simulink model "TableDeMiaxage"  (R2019a)
settings: Solver=VariableStepAuto  StartTime=0.0  StopTime=180  RelTol=1e-3
undefined symbols (not defined in the file): fdesignblkfcn, gcbh
libraries: dspvision x3, dspobslib x2, dspsrcs4 x1
settings Model: Creator=Ahmed  LastModifiedBy=shse

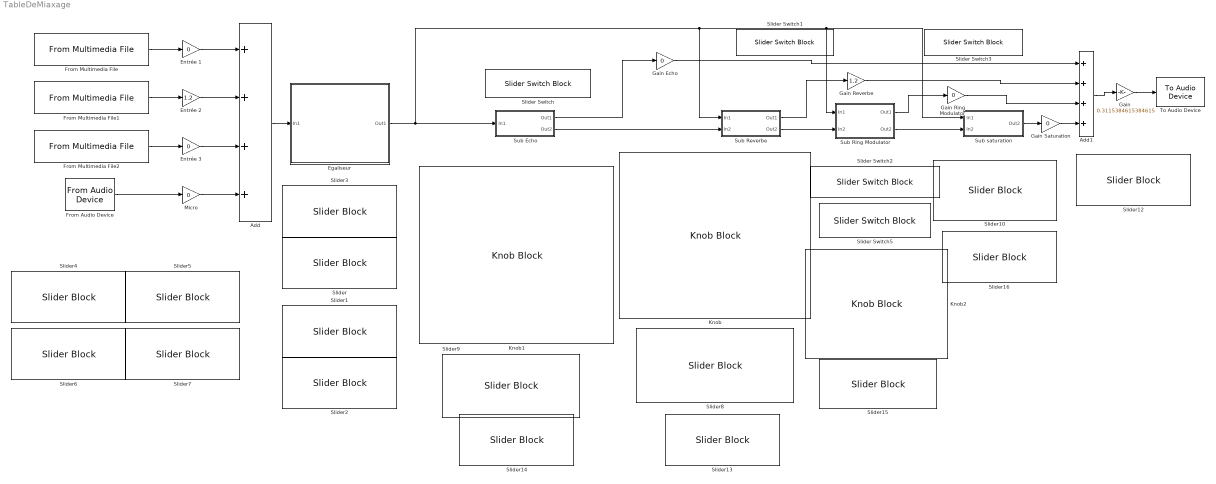
== system TableDeMiaxage ==
  Add : Sum  Inputs=++++
  Add1 : Sum  Inputs=++++
  Egaliseur : Subsystem
  Entrée 1 : Gain  Gain=0
  Entrée 2 : Gain  Gain=1.2
  Entrée 3 : Gain  Gain=0
  From Audio Device : dspobslib/From Audio Device  deviceName="Microphone (AT2020 USB               )"  numChannels=2  sampleRate=48000  deviceDatatype=Determine from output data type  autoBufferSize=on  bufferSize=4096  queueDuration=1.0  frameSize=1024  outputDatatype=double  defaultInputChannelMapping=on  inputChannelMapping=1:2  outputNumOverrunSamples=off  OutputFrames=on
      settings: SourceProductName=DSP System Toolbox  SourceProductBaseCode=DS
  From Multimedia File : dspvision/From Multimedia File  inputFilename=C:\Users\Ahmed\Nextcloud\L3\LU3EE105\Audio\Documents de TP et projet-20191118\Projet\because.wav  readRange=[1 Inf]  loop=on  numPlays=inf  outputStreams=Audio only  videoDataType=single  audioDataType=double  inheritSampleTime=on  userDefinedSampleTime=1/30  noAudioOutput=off  isIntensityVideo=off  fourcc=RGB  colorVideoFormat=Separate color signals  outputEOF=off  dataOrg=Column-major  audioFrameSize=1024  computeAudioFrameSize=off  outSamplingMode=Sample based
      settings: SourceProductName=DSP System Toolbox  SourceProductBaseCode=DS
  From Multimedia File1 : dspvision/From Multimedia File  inputFilename=C:\Users\Ahmed\Nextcloud\L3\LU3EE105\Audio\Documents de TP et projet-20191118\Projet\superstition.wav  readRange=[1 Inf]  loop=on  numPlays=inf  outputStreams=Audio only  videoDataType=single  audioDataType=double  inheritSampleTime=on  userDefinedSampleTime=1/30  noAudioOutput=off  isIntensityVideo=off  fourcc=RGB  colorVideoFormat=Separate color signals  outputEOF=off  dataOrg=Column-major  audioFrameSize=1024  computeAudioFrameSize=off  outSamplingMode=Sample based
      settings: SourceProductName=DSP System Toolbox  SourceProductBaseCode=DS
  From Multimedia File2 : dspvision/From Multimedia File  inputFilename=C:\Users\Ahmed\Nextcloud\L3\LU3EE105\Audio\Documents de TP et projet-20191118\Projet\tchai.wav  readRange=[1 Inf]  loop=on  numPlays=inf  outputStreams=Audio only  videoDataType=single  audioDataType=double  inheritSampleTime=on  userDefinedSampleTime=1/30  noAudioOutput=off  isIntensityVideo=off  fourcc=RGB  colorVideoFormat=Separate color signals  outputEOF=off  dataOrg=Column-major  audioFrameSize=1024  computeAudioFrameSize=off  outSamplingMode=Sample based
      settings: SourceProductName=DSP System Toolbox  SourceProductBaseCode=DS
  Gain : Gain  Gain=0.3115384615384615
  Gain Echo : Gain  Gain=0
  Gain Reverbe : Gain  Gain=1.2
  Gain Ring Modulator : Gain  Gain=0
  Gain Saturation : Gain  Gain=0
  Knob : KnobBlock  ScaleMax=48000
  Knob1 : KnobBlock  ScaleMax=48000
  Knob2 : KnobBlock  ScaleMin=100  ScaleMax=2000
  Micro : Gain  Gain=0
  Slider{,1..7} (8 alike) : SliderBlock  ScaleMax=1.2
  Slider Switch{,1..3,5} (5 alike) : SliderSwitchBlock
  Slider10 : SliderBlock  ScaleMax=1.5
  Slider12 : SliderBlock  ScaleMax=1.5
  Slider{13..16} (4 alike) : SliderBlock  ScaleMax=2
  Slider8 : SliderBlock  ScaleMax=1
  Slider9 : SliderBlock  ScaleMax=1
  Sub Echo : Subsystem
  Sub Reverbe : Subsystem
  Sub Ring Modulator : Subsystem
  Sub saturation : Subsystem
  To Audio Device : dspobslib/To Audio Device  deviceName=Default  inheritSampleRate=on  sampleRate=44100  deviceDatatype=Determine from input data type  autoBufferSize=on  bufferSize=4096  queueDuration=1.0  defaultOutputChannelMapping=on  outputChannelMapping=1:2  outputNumUnderrunSamples=off
      settings: SourceProductName=DSP System Toolbox  SourceProductBaseCode=DS
  wires:
  From Multimedia File/1 -> Entrée 1/1
  From Multimedia File1/1 -> Entrée 2/1
  From Multimedia File2/1 -> Entrée 3/1
  From Audio Device/1 -> Micro/1
  Micro/1 -> Add/4
  Entrée 3/1 -> Add/3
  Entrée 2/1 -> Add/2
  Entrée 1/1 -> Add/1
  Add/1 -> Egaliseur/1(In1)
  Add1/1 -> Gain/1
  Sub Reverbe/2(Out2) -> Sub Ring Modulator/2(In2)
  Sub Reverbe/1(Out1) -> Gain Reverbe/1
  Sub Echo/2(Out2) -> Sub Reverbe/2(In2)
  Egaliseur/1(Out1) -> Sub Reverbe/1(In1), Sub Ring Modulator/1(In1), Sub saturation/1(In1), Sub Echo/1(In1)
  Sub Echo/1(Out1) -> Gain Echo/1
  Gain/1 -> To Audio Device/1
  Sub saturation/1(Out2) -> Gain Saturation/1
  Sub Ring Modulator/2(Out2) -> Sub saturation/2(In2)
  Sub Ring Modulator/1(Out1) -> Gain Ring Modulator/1
  Gain Echo/1 -> Add1/1
  Gain Reverbe/1 -> Add1/2
  Gain Ring Modulator/1 -> Add1/3
  Gain Saturation/1 -> Add1/4

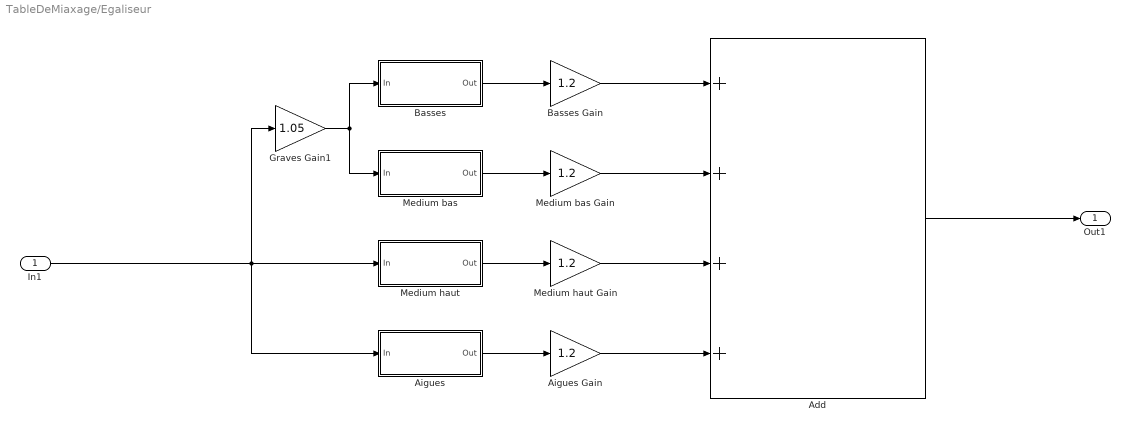
== system TableDeMiaxage/Egaliseur ==
  In1 : Inport
  Add : Sum  Inputs=++++
  Aigues : Subsystem  DialogController=fdesignblkfcn  InitFcn=fdesignblkfcn(gcbh, {'InitFcn'});  mask(Highpass Filter){}
      mask help: Design a highpass filter
      settings: CopyFcn=fdesignblkfcn(gcbh, {'CopyFcn'});
      mask Help: helpview(mapfilelocation('dsp'), 'dsphighpassfilter');
      mask Display: disp('Highpass')
  Aigues Gain : Gain  Gain=1.2
  Basses : Subsystem  DialogController=fdesignblkfcn  InitFcn=fdesignblkfcn(gcbh, {'InitFcn'});  mask(Lowpass Filter){}
      mask help: Design a lowpass filter
      settings: CopyFcn=fdesignblkfcn(gcbh, {'CopyFcn'});
      mask Help: helpview(mapfilelocation('dsp'), 'dsplowpassfilter');
      mask Display: disp('Lowpass')
  Basses Gain : Gain  Gain=1.2
  Graves Gain1 : Gain  Gain=1.05
  Medium bas : Subsystem  DialogController=fdesignblkfcn  InitFcn=fdesignblkfcn(gcbh, {'InitFcn'});  mask(Bandpass Filter){}
      mask help: Design a bandpass filter
      settings: CopyFcn=fdesignblkfcn(gcbh, {'CopyFcn'});
      mask Help: helpview(mapfilelocation('dsp'), 'dspbandpassfilter');
      mask Display: disp('Bandpass');
  Medium bas Gain : Gain  Gain=1.2
  Medium haut : Subsystem  DialogController=fdesignblkfcn  InitFcn=fdesignblkfcn(gcbh, {'InitFcn'});  mask(Bandpass Filter){}
      mask help: Design a bandpass filter
      settings: CopyFcn=fdesignblkfcn(gcbh, {'CopyFcn'});
      mask Help: helpview(mapfilelocation('dsp'), 'dspbandpassfilter');
      mask Display: disp('Bandpass');
  Medium haut Gain : Gain  Gain=1.2
  Out1 : Outport
  wires:
  Graves Gain1/1 -> Basses/1(In), Medium bas/1(In)
  Add/1 -> Out1/1
  Aigues Gain/1 -> Add/4
  Medium haut Gain/1 -> Add/3
  Medium bas/1(Out) -> Medium bas Gain/1
  Medium bas Gain/1 -> Add/2
  Basses Gain/1 -> Add/1
  Basses/1(Out) -> Basses Gain/1
  In1/1 -> Aigues/1(In), Medium haut/1(In), Graves Gain1/1
  Medium haut/1(Out) -> Medium haut Gain/1
  Aigues/1(Out) -> Aigues Gain/1

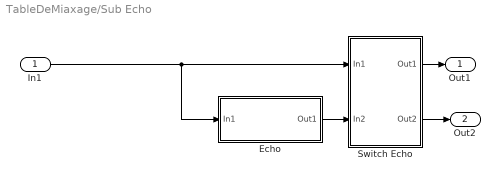
== system TableDeMiaxage/Sub Echo ==
  In1 : Inport
  Echo : Subsystem
  Switch Echo : Subsystem
  Out1 : Outport
  Out2 : Outport  Port=2
  wires:
  Echo/1(Out1) -> Switch Echo/2(In2)
  Switch Echo/1(Out1) -> Out1/1
  In1/1 -> Echo/1(In1), Switch Echo/1(In1)
  Switch Echo/2(Out2) -> Out2/1

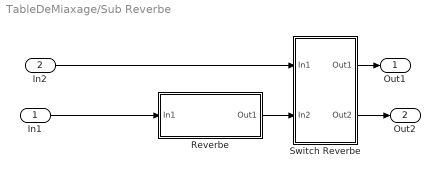
== system TableDeMiaxage/Sub Reverbe ==
  In1 : Inport
  In2 : Inport  Port=2
  Reverbe : Subsystem
  Switch Reverbe : Subsystem
  Out1 : Outport
  Out2 : Outport  Port=2
  wires:
  In1/1 -> Reverbe/1(In1)
  Reverbe/1(Out1) -> Switch Reverbe/2(In2)
  In2/1 -> Switch Reverbe/1(In1)
  Switch Reverbe/2(Out2) -> Out2/1
  Switch Reverbe/1(Out1) -> Out1/1

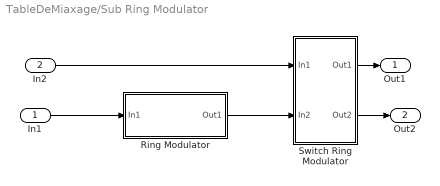
== system TableDeMiaxage/Sub Ring Modulator ==
  In1 : Inport
  In2 : Inport  Port=2
  Ring Modulator : Subsystem
  Switch Ring Modulator : Subsystem
  Out1 : Outport
  Out2 : Outport  Port=2
  wires:
  In1/1 -> Ring Modulator/1(In1)
  Ring Modulator/1(Out1) -> Switch Ring Modulator/2(In2)
  In2/1 -> Switch Ring Modulator/1(In1)
  Switch Ring Modulator/2(Out2) -> Out2/1
  Switch Ring Modulator/1(Out1) -> Out1/1

== system TableDeMiaxage/Sub saturation ==
  In1 : Inport
  In2 : Inport  Port=2
  Switch saturation : Subsystem
  saturation : Subsystem
  Out2 : Outport
  wires:
  In1/1 -> saturation/1(In1)
  saturation/1(Out1) -> Switch saturation/2(In2)
  In2/1 -> Switch saturation/1(In1)
  Switch saturation/1(Out2) -> Out2/1

== system TableDeMiaxage/Egaliseur/Aigues ==
  In : Inport
  Generated Filter Block : DiscreteFir  Tag=BlockMethodSubSystem  Coefficients=[0.0167926706972023297 -0.00307522082859672382 -0.00155836801096264905 0.00678688212494691322 -0.00921947504734154516 0.00716180335937461818 -0.00202417819565003281 -0.00247958884121546579 0.00297471068413305249 0.000980534073277820146 -0.00634024282569068624 0.00870304843048571274 -0.00569033146091242701 -0.000974243416099627264 0.00644942423308224929 -0.00633706852781140001 0.000239642776776960632 0.00749483357856131193 -0.0107451066385319625 0.00631082658742477751 0.00317079948780857714 -0.0107615026768319855 0.0101264166919688165 -0.000871435749622451617 -0.0105995290115455873 0.0152814722852097698 -0.00843240688530845495 -0.00602945332444454647 0.0174768179112361685 -0.016173414015238835 0.00118274129148582654 0.0175174930605758797 -0.0252362821856293232 0.0134963666514811807 0.0120367581497580443 -0.0332563662689180084 0.0313194480469127026 -0.00133439181794675599 -0.0402321887557888502 0.0620015888628606057 -0.0357204359625284198 -0.044553870224684676 0.154599277267642304 -0.249627721101705446 0.287093803988040797 -0.249627721101705446 0.154599277267642304 -0.044553870224684676 -0.0357204359625284198 0.0620015888628606057 -0.0402321887557888502 -0.00133439181794675599 0.0313194480469127026 -0.0332563662689180084 0.0120367581497580443 0.0134963666514811807 -0.0252362821856293232 0.0175174930605758797 0.00118274129148582654 -0.016173414015238835 0.0174768179112361685 -0.00602945332444454647 -0.00843240688530845495 0.0152814722852097698 -0.0105995290115455873 -0.000871435749622451617 0.0101264166919688165 -0.0107615026768319855 0.00317079948780857714 0.00631082658742477751 -0.0107451066385319625 0.00749483357856131193 0.000239642776776960632 -0.00633706852781140001 0.00644942423308224929 -0.000974243416099627264 -0.00569033146091242701 0.00870304843048571274 -0.00634024282569068624 0.000980534073277820146 0.00297471068413305249 -0.00247958884121546579 -0.00202417819565003281 0.00716180335937461818 -0.00921947504734154516 0.00678688212494691322 -0.00155836801096264905 -0.00307522082859672382 0.0167926706972023297]  InputProcessing=Columns as channels (frame based)
  Out : Outport
  wires:
  In/1 -> Generated Filter Block/1
  Generated Filter Block/1 -> Out/1

== system TableDeMiaxage/Egaliseur/Basses ==
  In : Inport
  Generated Filter Block : DiscreteFir  Tag=BlockMethodSubSystem  Coefficients=[-0.0153884254991570896 0.000266804767962262673 0.000327964912984287542 0.000425773956292074178 0.000562470431597255683 0.000729675436245145743 0.000928098732682747078 0.00114757496934848988 0.0013874893535819144 0.00163674485373585228 0.00189397943095723415 0.00214911176559310756 0.00239127376957799917 0.00261871580170263676 0.00282463549794394458 0.00299796194879956577 0.00313700441606081177 0.00323118901775356227 0.00328059593937512052 0.0032762274085140616 0.00321999924325729308 0.00310514488595467486 0.00293597620135533548 0.00271021313991444326 0.00243244432834343769 0.00210285539361005757 0.00173075814627612814 0.00131794874767348713 0.000876458309185095593 0.000409765769008486587 -6.78152181175429349e-05 -0.00055107827022111359 -0.00102452357018295213 -0.00148228311788735465 -0.00190917788438955548 -0.00229835807769330699 -0.00263554870259227183 -0.00291558267477844222 -0.00312595002418917817 -0.00326368850063736733 -0.0033181487660765268 -0.00329019210437426091 -0.00317265655073278429 -0.00297008708884775961 -0.00267912961982578503 -0.00230819118685900767 -0.00185871380492080222 -0.00134285673590555732 -0.000766282213175846516 -0.000143639886938228738 0.000515387431471188277 0.00119186250405529915 0.00187540925341580437 0.00254498623467350367 0.00318890021840806609 0.00378542058067834163 0.00432300298736445088 0.00478127017511513746 0.00515003046032541049 0.00541280250324055381 0.00555799365296140262 0.00557670671392240021 0.00546500919878054655 0.00521345698067954538 0.0048255975064855107 0.00429822188412450328 0.00364138491650149547 0.00285830087950445259 0.00196522256851390346 0.000971608832914958248 -0.000117014335600230956 -0.00121216225006984778 -0.00238215104275762242 -0.00356276040555317426 -0.00472456049283136344 -0.0058457030770970005 -0.00689286435319730502 -0.00784296295490719345 -0.00866238471873602076 -0.00932881033341804826 -0.00981062820326479915 -0.0100871412549760533 -0.0101477740694355528 -0.00995366092214836767 -0.00949962887211590855 -0.00877727431061372382 -0.00777478005111272019 -0.00649472069378163788 -0.0049340887119306712 -0.0031050204118294694 -0.0010140823683356785 0.0013172912006325472 0.00387347512217753364 0.00662624416734313923 0.00954783933336443569 0.0126033841210471554 0.015761493515271157 0.0189793379213840825 0.022221591185954695 0.025441734970274868 0.0286029070172382494 0.0316580472453209458 0.0345709721826798211 0.0372966552097049875 0.039801977564689818 0.0420483051028727392 0.0440079277575662273 0.0456487202321445365 0.0469517485160680023 0.0478939985283200892 0.0484669205309821716 0.0486571254135078901 0.0484669205309821716 0.0478939985283200892 0.0469517485160680023 0.0456487202321445365 0.0440079277575662273 0.0420483051028727392 0.039801977564689818 0.0372966552097049875 0.0345709721826798211 0.0316580472453209458 0.0286029070172382494 0.025441734970274868 0.022221591185954695 0.0189793379213840825 0.015761493515271157 0.0126033841210471554 0.00954783933336443569 0.00662624416734313923 0.00387347512217753364 0.0013172912006325472 -0.0010140823683356785 -0.0031050204118294694 -0.0049340887119306712 -0.00649472069378163788 -0.00777478005111272019 -0.00877727431061372382 -0.00949962887211590855 -0.00995366092214836767 -0.0101477740694355528 -0.0100871412549760533 -0.00981062820326479915 -0.00932881033341804826 -0.00866238471873602076 -0.00784296295490719345 -0.00689286435319730502 -0.0058457030770970005 -0.00472456049283136344 -0.00356276040555317426 -0.00238215104275762242 -0.00121216225006984778 -0.000117014335600230956 0.000971608832914958248 0.00196522256851390346 0.00285830087950445259 0.00364138491650149547 0.00429822188412450328 0.0048255975064855107 0.00521345698067954538 0.00546500919878054655 0.00557670671392240021 0.00555799365296140262 0.00541280250324055381 0.00515003046032541049 0.00478127017511513746 0.00432300298736445088 0.00378542058067834163 0.00318890021840806609 0.00254498623467350367 0.00187540925341580437 0.00119186250405529915 0.000515387431471188277 ...(+1178 chars)]  InputProcessing=Columns as channels (frame based)
  Out : Outport
  wires:
  Generated Filter Block/1 -> Out/1
  In/1 -> Generated Filter Block/1

== system TableDeMiaxage/Egaliseur/Medium bas ==
  In : Inport
  Generated Filter Block : DiscreteFir  Tag=BlockMethodSubSystem  Coefficients=[0.0140352068792694695 -0.0026321581708315606 -0.00197079210321328673 -0.00106112498534715119 0.000119472592524640664 0.00149628691001717456 0.00288950002374261132 0.00403507302723793339 0.00462865274118079689 0.00442403000305877179 0.0033086518772103635 0.00138267709792085167 -0.00104985853714803035 -0.0035210229224174926 -0.00552832551549370735 -0.00665115471996120377 -0.00668714826848286568 -0.00569744778503787196 -0.00401379410865280745 -0.00213152434676947217 -0.000587866401658069799 0.000211313099421048923 9.26059013533169612e-05 -0.000816071422381474767 -0.00214443357310104173 -0.00337786798559317836 -0.00403814902921402659 -0.00381763639679466712 -0.00269745217172421116 -0.000937812781028578507 0.000984490769474923857 0.00254680327966371389 0.00333221532232293345 0.003187161448757666 0.00225869715921652153 0.00097075945933320707 -0.000130077018285688402 -0.000537319876968455181 2.21341188739474442e-05 0.00150269518925763351 0.00351917039302384726 0.00547575758577071962 0.00673241554142266826 0.00683180879036704783 0.00563850632989189565 0.00341743817076089378 0.000746660718113200316 -0.00163762705736385738 -0.00309259568193187865 -0.00326192031958997706 -0.00222142721037315617 -0.000450783745724910002 0.00129031609662780028 0.00222197460493422884 0.00178417455709858376 -0.000145393726253772841 -0.00320497685551981298 -0.00662011660068355726 -0.00945198334806177792 -0.01087295383788431 -0.0104577619984935841 -0.00831894631182310447 -0.00511204885286287332 -0.00182568010578164179 0.000508414278906465307 0.00117162998769634289 -8.88496532107276473e-06 -0.00255649427792050939 -0.00548789393078537302 -0.00759185611198433599 -0.00783726957197261771 -0.00570725546554719763 -0.00142332272859732882 0.00409671810021271926 0.00947149062392063819 0.0132917971445410104 0.0145527259605028395 0.0130186027776133337 0.00932127126199720768 0.00482015957386658887 0.00117754685766334986 -0.000154667691669789709 0.00154720377882020259 0.0060006138912535251 0.0119085230015501531 0.0173195036305196469 0.0201904251324107539 0.0190626229695590767 0.0135669404687462237 0.0046588650376496489 -0.00558981351746895734 -0.0145376995349663484 -0.0197907573344304893 -0.0199792654490850187 -0.0153222643270756222 -0.00770748748605236227 -0.000290727845660914514 0.00338439876908689817 0.000452543286244571957 -0.0102477027132580282 -0.0275684229641616069 -0.0480126044915529099 -0.0663981915494953473 -0.0770356306832355869 -0.075206854390709621 -0.0585017928200668516 -0.0277050936146285218 0.0130893398667307759 0.0571605795622653831 0.0965439388183477881 0.123777652180148454 0.13345175363554565 0.123777652180148454 0.0965439388183477881 0.0571605795622653831 0.0130893398667307759 -0.0277050936146285218 -0.0585017928200668516 -0.075206854390709621 -0.0770356306832355869 -0.0663981915494953473 -0.0480126044915529099 -0.0275684229641616069 -0.0102477027132580282 0.000452543286244571957 0.00338439876908689817 -0.000290727845660914514 -0.00770748748605236227 -0.0153222643270756222 -0.0199792654490850187 -0.0197907573344304893 -0.0145376995349663484 -0.00558981351746895734 0.0046588650376496489 0.0135669404687462237 0.0190626229695590767 0.0201904251324107539 0.0173195036305196469 0.0119085230015501531 0.0060006138912535251 0.00154720377882020259 -0.000154667691669789709 0.00117754685766334986 0.00482015957386658887 0.00932127126199720768 0.0130186027776133337 0.0145527259605028395 0.0132917971445410104 0.00947149062392063819 0.00409671810021271926 -0.00142332272859732882 -0.00570725546554719763 -0.00783726957197261771 -0.00759185611198433599 -0.00548789393078537302 -0.00255649427792050939 -8.88496532107276473e-06 0.00117162998769634289 0.000508414278906465307 -0.00182568010578164179 -0.00511204885286287332 -0.00831894631182310447 -0.0104577619984935841 -0.01087295383788431 -0.00945198334806177792 -0.00662011660068355726 -0.00320497685551981298 -0.000145393726253772841 0.00178417455709858376 0.00222197460493422884 0.00129031609662780028 -0.000450783745724910002 ...(+1203 chars)]  InputProcessing=Columns as channels (frame based)
  Out : Outport
  wires:
  Generated Filter Block/1 -> Out/1
  In/1 -> Generated Filter Block/1

== system TableDeMiaxage/Egaliseur/Medium haut ==
  In : Inport
  Generated Filter Block : DiscreteFir  Tag=BlockMethodSubSystem  Coefficients=[-0.0062414651454274642 0.00389811490713546207 -0.00280397911484692522 0.0174041899535088453 0.0150234854508142345 -0.00795848740988005718 -0.00309119797675585367 0.00355535780647063798 -0.00735420524198353992 -0.00288182443407250695 0.000158523985061867457 -0.00304210584932094888 0.00545473828870900266 0.00328135450605069419 0.00146139947744780541 0.0078168453579246476 -0.00138536693675637089 -0.00264907845512550848 0.000864050116544914665 -0.00951359554714665753 -0.00382578749104094725 0.000509686093973454857 -0.00569312592864624264 0.00663342842314541044 0.00681976104846186357 0.000565813629693356131 0.0107921924262149357 0.00042835263422412326 -0.00607710948205151917 0.00183321306791148545 -0.0122104718903303898 -0.00857456861614619946 0.00264988750831648707 -0.00784110215030565764 0.00697549514369134177 0.0134313646205669983 -5.8583941705461682e-05 0.0141909752630037765 0.00457496837846286652 -0.0121757201035912945 0.00209347277353455702 -0.0152414310377332555 -0.017999628925225452 0.00574833807160543726 -0.00969720498516807479 0.0060072035281790578 0.0264653467152446663 0.000707804499679243974 0.0187677252195765573 0.0145026148781668036 -0.0243539020453497519 -0.000448621907164989463 -0.0202526630991497099 -0.0415967417835283737 0.0107546240370999264 -0.0109754289930505261 0.00173192691052212336 0.0662486970342087006 0.00932202145947663881 0.0325530498318659101 0.0573490960813152484 -0.0792038809701490626 -0.0270061826842571476 -0.0573703721449224588 -0.300220108539047681 0.0755662256194030713 0.534024536814492135 0.0755662256194030713 -0.300220108539047681 -0.0573703721449224588 -0.0270061826842571476 -0.0792038809701490626 0.0573490960813152484 0.0325530498318659101 0.00932202145947663881 0.0662486970342087006 0.00173192691052212336 -0.0109754289930505261 0.0107546240370999264 -0.0415967417835283737 -0.0202526630991497099 -0.000448621907164989463 -0.0243539020453497519 0.0145026148781668036 0.0187677252195765573 0.000707804499679243974 0.0264653467152446663 0.0060072035281790578 -0.00969720498516807479 0.00574833807160543726 -0.017999628925225452 -0.0152414310377332555 0.00209347277353455702 -0.0121757201035912945 0.00457496837846286652 0.0141909752630037765 -5.8583941705461682e-05 0.0134313646205669983 0.00697549514369134177 -0.00784110215030565764 0.00264988750831648707 -0.00857456861614619946 -0.0122104718903303898 0.00183321306791148545 -0.00607710948205151917 0.00042835263422412326 0.0107921924262149357 0.000565813629693356131 0.00681976104846186357 0.00663342842314541044 -0.00569312592864624264 0.000509686093973454857 -0.00382578749104094725 -0.00951359554714665753 0.000864050116544914665 -0.00264907845512550848 -0.00138536693675637089 0.0078168453579246476 0.00146139947744780541 0.00328135450605069419 0.00545473828870900266 -0.00304210584932094888 0.000158523985061867457 -0.00288182443407250695 -0.00735420524198353992 0.00355535780647063798 -0.00309119797675585367 -0.00795848740988005718 0.0150234854508142345 0.0174041899535088453 -0.00280397911484692522 0.00389811490713546207 -0.0062414651454274642]  InputProcessing=Columns as channels (frame based)
  Out : Outport
  wires:
  Generated Filter Block/1 -> Out/1
  In/1 -> Generated Filter Block/1

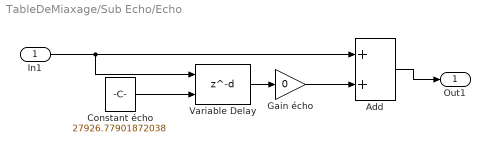
== system TableDeMiaxage/Sub Echo/Echo ==
  In1 : Inport
  Add : Sum
  Constant écho : Constant  Value=27926.77901872038  VectorParams1D=off
  Gain écho : Gain  Gain=0
  Variable Delay : Delay  DelayLengthSource=Input port  DelayLength=1  DelayLengthUpperLimit=5000  PreventDirectFeedthrough=on  RemoveDelayLengthCheckInGeneratedCode=on  InputProcessing=Columns as channels (frame based)
      settings: InputPortMap=u0,p1
  Out1 : Outport
  wires:
  In1/1 -> Variable Delay/1, Add/1
  Constant écho/1 -> Variable Delay/2
  Variable Delay/1 -> Gain écho/1
  Gain écho/1 -> Add/2
  Add/1 -> Out1/1

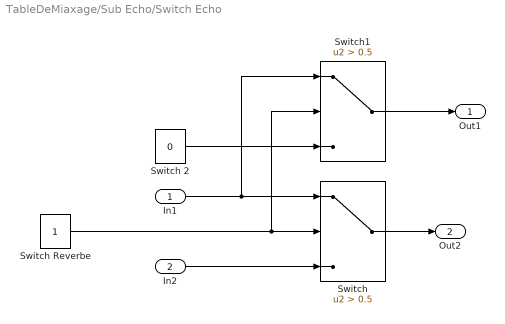
== system TableDeMiaxage/Sub Echo/Switch Echo ==
  In1 : Inport
  In2 : Inport  Port=2
  Switch : Switch  Criteria=u2 > Threshold  Threshold=0.5
  Switch 2 : Constant  Value=0  VectorParams1D=off
  Switch Reverbe : Constant  VectorParams1D=off
  Switch1 : Switch  Criteria=u2 > Threshold  Threshold=0.5
  Out1 : Outport
  Out2 : Outport  Port=2
  wires:
  In2/1 -> Switch/3
  In1/1 -> Switch1/1, Switch/1
  Switch/1 -> Out2/1
  Switch Reverbe/1 -> Switch/2, Switch1/2
  Switch 2/1 -> Switch1/3
  Switch1/1 -> Out1/1

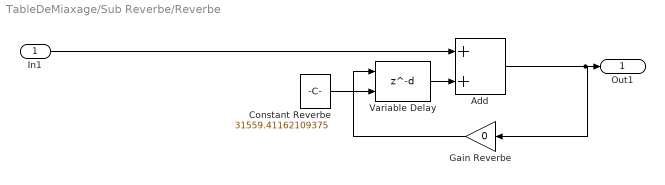
== system TableDeMiaxage/Sub Reverbe/Reverbe ==
  In1 : Inport
  Add : Sum
  Constant Reverbe : Constant  Value=31559.41162109375  VectorParams1D=off
  Gain Reverbe : Gain  Gain=0
  Variable Delay : Delay  DelayLengthSource=Input port  DelayLength=1  DelayLengthUpperLimit=5000  PreventDirectFeedthrough=on  RemoveDelayLengthCheckInGeneratedCode=on  InputProcessing=Columns as channels (frame based)
      settings: InputPortMap=u0,p1
  Out1 : Outport
  wires:
  Constant Reverbe/1 -> Variable Delay/2
  Gain Reverbe/1 -> Variable Delay/1
  Add/1 -> Out1/1, Gain Reverbe/1
  In1/1 -> Add/1
  Variable Delay/1 -> Add/2

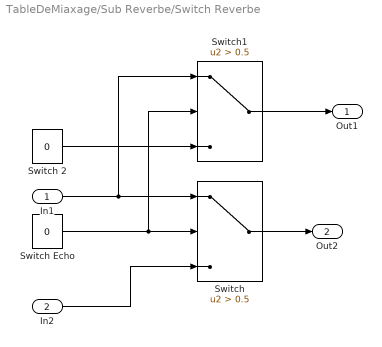
== system TableDeMiaxage/Sub Reverbe/Switch Reverbe ==
  In1 : Inport
  In2 : Inport  Port=2
  Switch : Switch  Criteria=u2 > Threshold  Threshold=0.5
  Switch 2 : Constant  Value=0  VectorParams1D=off
  Switch Echo : Constant  Value=0  VectorParams1D=off
  Switch1 : Switch  Criteria=u2 > Threshold  Threshold=0.5
  Out1 : Outport
  Out2 : Outport  Port=2
  wires:
  Switch 2/1 -> Switch1/3
  Switch/1 -> Out2/1
  In1/1 -> Switch1/1, Switch/1
  In2/1 -> Switch/3
  Switch1/1 -> Out1/1
  Switch Echo/1 -> Switch/2, Switch1/2

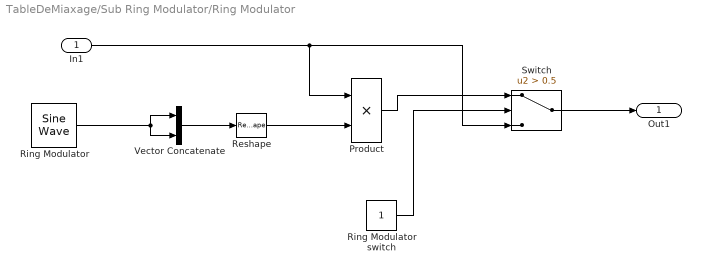
== system TableDeMiaxage/Sub Ring Modulator/Ring Modulator ==
  In1 : Inport
  Product : Product
  Reshape : Reshape  OutputDimensionality=Customize  OutputDimensions=[1024,2]
  Ring Modulator : dspsrcs4/Sine Wave  Amplitude=1  Frequency=626.4678039550781  Phase=0  SampleMode=Discrete  OutComplex=Real  CompMethod=Trigonometric fcn  TableSize=Speed  SampleTime=1/48000  SamplesPerFrame=1024  ResetState=Restart at time zero  OutputFrames=off  dataType=double  wordLen=16  udDataType=sfix(16)  fracBitsMode=Best precision  numFracBits=15  OutDataTypeStr=double  LastOutDataTypeStr=double
  Ring Modulator switch : Constant
  Switch : Switch  Criteria=u2 > Threshold  Threshold=0.5
  Vector Concatenate : Concatenate
  Out1 : Outport
  wires:
  Ring Modulator/1 -> Vector Concatenate/2, Vector Concatenate/1
  Reshape/1 -> Product/2
  Vector Concatenate/1 -> Reshape/1
  Ring Modulator switch/1 -> Switch/2
  Product/1 -> Switch/1
  In1/1 -> Product/1, Switch/3
  Switch/1 -> Out1/1

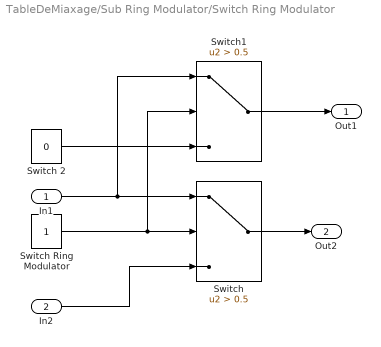
== system TableDeMiaxage/Sub Ring Modulator/Switch Ring Modulator ==
  In1 : Inport
  In2 : Inport  Port=2
  Switch : Switch  Criteria=u2 > Threshold  Threshold=0.5
  Switch 2 : Constant  Value=0  VectorParams1D=off
  Switch Ring Modulator : Constant  VectorParams1D=off
  Switch1 : Switch  Criteria=u2 > Threshold  Threshold=0.5
  Out1 : Outport
  Out2 : Outport  Port=2
  wires:
  Switch 2/1 -> Switch1/3
  Switch/1 -> Out2/1
  In1/1 -> Switch1/1, Switch/1
  In2/1 -> Switch/3
  Switch1/1 -> Out1/1
  Switch Ring Modulator/1 -> Switch/2, Switch1/2

== system TableDeMiaxage/Sub saturation/Switch saturation ==
  In1 : Inport
  In2 : Inport  Port=2
  Switch : Switch  Criteria=u2 > Threshold  Threshold=0.5
  Switch saturation : Constant  Value=0  VectorParams1D=off
  Out2 : Outport
  wires:
  Switch/1 -> Out2/1
  In1/1 -> Switch/1
  In2/1 -> Switch/3
  Switch saturation/1 -> Switch/2

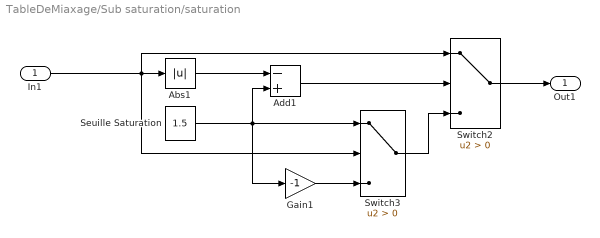
== system TableDeMiaxage/Sub saturation/saturation ==
  In1 : Inport
  Abs1 : Abs
  Add1 : Sum  Inputs=-+
  Gain1 : Gain  Gain=-1
  Seuille Saturation : Constant  Value=1.5  VectorParams1D=off
  Switch2 : Switch  Criteria=u2 > Threshold
  Switch3 : Switch  Criteria=u2 > Threshold
  Out1 : Outport
  wires:
  Switch3/1 -> Switch2/3
  In1/1 -> Abs1/1, Switch3/2, Switch2/1
  Gain1/1 -> Switch3/3
  Switch2/1 -> Out1/1
  Abs1/1 -> Add1/1
  Add1/1 -> Switch2/2
  Seuille Saturation/1 -> Add1/2, Switch3/1, Gain1/1
